simulink model "transfer_function_calculation"  (R2016a)
settings: Solver=VariableStepAuto  StartTime=0.0  StopTime=5  RelTol=1e-3
values from neighbouring files (symbols this model uses):
  a = .7    (= 0.7)    [PM_1_5MW_syn_27.m]
  Flux = 5.8264    [PM_1_5MW_syn_27.m]
  Id_set = 500    [PM_1_5MW_syn_27.m]
  Iq_set = -2200    [PM_1_5MW_syn_27.m]
  L = .0001    (= 0.0001)    [PM_1_5MW_syn_27.m]
  Ld = 0.001575    [PM_1_5MW_syn_27.m]
  Lq = 0.001575    [PM_1_5MW_syn_27.m]
  mn = 60000    [PM_1_5MW_syn_27.m]
  p = 26    [PM_1_5MW_syn_27.m]
  Rs = 0.000821    [PM_1_5MW_syn_27.m]
  Sollkurve_M_Optimum = [0 57121 101549 158670 228485 310994 406196 514092 634681 767965 810425 823386 ... (13 elements, 13x1)]    [Lookup_M_n.mat]
  Sollkurve_nGen_Optimum = [0 5 7 9 11 12 14 16 18 20 20.07 20.2 ... (13 elements, 13x1)]    [Lookup_M_n.mat]
  Speed_set = w_m    (= 2.10172548525)    [PM_1_5MW_syn_27.m]
  Ts_Power = 5.000000000000000e-06    (= 5e-06)    [PM_1_5MW_syn_27.m]
  Vdc = 1200    [PM_1_5MW_syn_27.m]
  Vh = Vm/6*0    (= 0)    [PM_1_5MW_syn_27.m]
undefined symbols (not defined in the file or in its folder): C2, Esw_Erec, Esw_Off, Esw_On, Page_Temp_C
undefined symbols (not defined in the file): Ts_Control, z
libraries: fl_lib x84, powerlib_meascontrol x58, simulink x56, nesl_utility x36, powerlib x33, simulink_extras x11
(part 1 of 6)
settings Model: Creator=Test  LastModifiedBy=Test

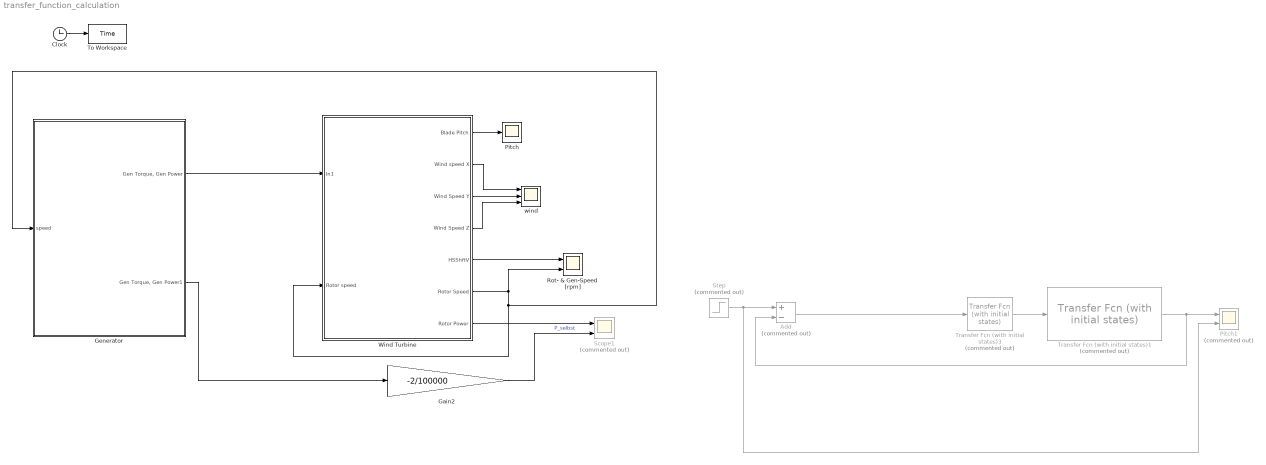
== system transfer_function_calculation ==
  Add : Sum  Commented=on  Inputs=+-
  Clock : Clock
  Gain2 : Gain  Gain=-2/100000
  Generator : Subsystem
  Pitch : Scope
  Pitch1 : Scope  Commented=on  NumInputPorts=2
  Rot- & Gen-Speed [rpm] : Scope  NumInputPorts=2
  Scope1 : Scope  Commented=on  NumInputPorts=2
  Step : Step  Commented=on  SampleTime=0
  To Workspace : ToWorkspace  VariableName=Time  SampleTime=-1
  Transfer Fcn (with initial states)1 : simulink_extras/Additional Linear/Transfer Fcn (with initial states)  Commented=on  N=[6349]  D=[1 10.52 5.213]  X0=0
  Transfer Fcn (with initial states)3 : simulink_extras/Additional Linear/Transfer Fcn (with initial states)  Commented=on  N=[-627e-6 1]*5  D=[627e-6 1]  X0=0
  Wind Turbine : Subsystem
  wind : Scope  NumInputPorts=3
  wires:
  Clock/1 -> To Workspace/1
  Generator/2("Gen Torque, Gen Power1") -> Gain2/1
  Gain2/1 -> Scope1/2  "P_selbst"
  Wind Turbine/6(Rotor Speed) -> Generator/1(speed), Wind Turbine/2(Rotor speed), Rot- & Gen-Speed [rpm]/2
  Generator/1("Gen Torque, Gen Power") -> Wind Turbine/1(In1)
  Wind Turbine/1(Blade Pitch) -> Pitch/1
  Wind Turbine/2(Wind speed X) -> wind/1
  Wind Turbine/3(Wind Speed Y) -> wind/2
  Wind Turbine/4(Wind Speed Z) -> wind/3
  Wind Turbine/7(Rotor Power) -> Scope1/1
  Wind Turbine/5(HSShftV) -> Rot- & Gen-Speed [rpm]/1
  Transfer Fcn (with initial states)1/1 -> Add/2, Pitch1/1
  Step/1 -> Pitch1/2, Add/1
  Add/1 -> Transfer Fcn (with initial states)3/1
  Transfer Fcn (with initial states)3/1 -> Transfer Fcn (with initial states)1/1

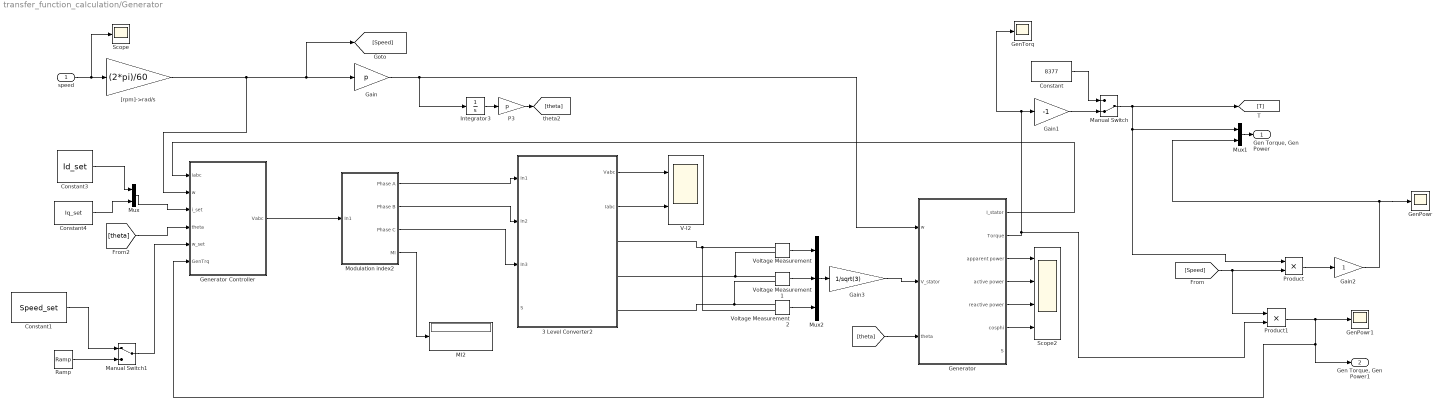
== system transfer_function_calculation/Generator ==
  speed : Inport
  3 Level Converter2 : Subsystem
  Constant : Constant  Value=8377  VectorParams1D=off
  Constant1 : Constant  Value=Speed_set  VectorParams1D=off
  Constant3 : Constant  Value=Id_set
  Constant4 : Constant  Value=Iq_set
  Gain : Gain  Gain=p
  Gain1 : Gain  Gain=-1
  Gain2 : Gain
  Gain3 : Gain  Gain=1/sqrt(3)
  GenPowr : Scope
  GenPowr1 : Scope
  GenTorq : Scope
  "Generator " : Subsystem
  "Generator Controller " : Subsystem
  Integrator3 : Integrator
  MI2 : Display
  Manual Switch : ManualSwitch  CurrentSetting=0
  Manual Switch1 : ManualSwitch
  Modulation index2 : Subsystem
  Mux : Mux  Inputs=2
  Mux1 : Mux  Inputs=2
  Mux2 : Mux  Inputs=3
  P3 : Gain  Gain=p
  Product : Product
  Product1 : Product
  Ramp : simulink/Sources/Ramp  slope=1/60*2*pi/10  start=40  X0=1.831548517042849
  Scope : Scope
  Scope2 : Scope  NumInputPorts=4
  V-I2 : Scope  NumInputPorts=2
  Voltage Measurement : powerlib/Measurements/Voltage Measurement  PhasorSimulation=off  OutputType=Complex  PSBequivalent=0
  Voltage Measurement1 : powerlib/Measurements/Voltage Measurement  PhasorSimulation=off  OutputType=Complex  PSBequivalent=0
  Voltage Measurement2 : powerlib/Measurements/Voltage Measurement  PhasorSimulation=off  OutputType=Complex  PSBequivalent=0
  "[rpm]->rad/s" : Gain  Gain=(2*pi)/60
  "Gen Torque, Gen Power" : Outport
  "Gen Torque, Gen Power1" : Outport  Port=2
  wires:
  speed/1 -> "[rpm]->rad/s"/1, Scope/1
  "Generator "/1("I_stator ") -> "Generator Controller "/1(iabc)
  Constant3/1 -> Mux/1
  "Generator "/5(reactive power) -> Scope2/3
  [theta] -> "Generator Controller "/4(theta)
  Constant4/1 -> Mux/2
  "Generator "/6(cosphi) -> Scope2/4
  "Generator "/3(apparent power) -> Scope2/1
  "Generator "/4(active power) -> Scope2/2
  Constant1/1 -> Manual Switch1/1
  [theta] -> "Generator "/3("theta ")
  Mux/1 -> "Generator Controller "/3(i_set)
  Gain/1 -> "Generator "/1(w), Integrator3/1
  "[rpm]->rad/s"/1 -> "Generator Controller "/2(w), [Speed], Gain/1
  Integrator3/1 -> P3/1
  [Speed] -> Product/2, Product1/1
  Product1/1 -> "Generator Controller "/6(GenTrq), "Gen Torque, Gen Power1"/1, GenPowr1/1
  Mux1/1 -> "Gen Torque, Gen Power"/1
  Product/1 -> Gain2/1
  Constant/1 -> Manual Switch/1
  Gain2/1 -> GenPowr/1, Mux1/2
  "Generator "/2(Torque) -> GenTorq/1, Gain1/1, Product1/2
  Manual Switch/1 -> [T], Mux1/1, Product/1
  Manual Switch1/1 -> "Generator Controller "/5(w_set)
  Ramp/1 -> Manual Switch1/2
  Gain1/1 -> Manual Switch/2
  P3/1 -> [theta]
  3 Level Converter2/2(Iabc) -> V-I2/2
  Modulation index2/1(Phase A) -> 3 Level Converter2/1(In1)
  Modulation index2/2(Phase B) -> 3 Level Converter2/2(In2)
  Modulation index2/3(Phase C) -> 3 Level Converter2/3(In3)
  Modulation index2/4(MI) -> MI2/1
  3 Level Converter2/1(Vabc) -> V-I2/1
  Voltage Measurement/1 -> Mux2/1
  Voltage Measurement1/1 -> Mux2/2
  Voltage Measurement2/1 -> Mux2/3
  Mux2/1 -> Gain3/1
  Gain3/1 -> "Generator "/2("V_stator ")
  "Generator Controller "/1(Vabc) -> Modulation index2/1(In1)
  connections:
  Voltage Measurement/LConn1 -- Voltage Measurement2/LConn2 -- 3 Level Converter2/RConn1
  Voltage Measurement1/LConn1 -- Voltage Measurement/LConn2 -- 3 Level Converter2/RConn2
  Voltage Measurement2/LConn1 -- Voltage Measurement1/LConn2 -- 3 Level Converter2/RConn3

== system transfer_function_calculation/Wind Turbine ==
  In1 : Inport
  Rotor speed : Inport  Port=2
  FAST Nonlinear Wind Turbine : Subsystem  mask(FAST Nonlinear Wind Turbine){}
      mask help: This block contains the FAST S-Function.
      mask init:
      | clear FAST_SFunc
  High-Speed Shaft Brake : Subsystem
  Pitch Controller : Subsystem
  "Turbine Output Scope " : Subsystem
  Yaw Controller : Subsystem
  Blade Pitch : Outport
  Wind speed X : Outport  Port=2
  Wind Speed Y : Outport  Port=3
  Wind Speed Z : Outport  Port=4
  HSShftV : Outport  Port=5
  Rotor Speed : Outport  Port=6
  Rotor Power : Outport  Port=7
  wires:
  Pitch Controller/1(Out1) -> FAST Nonlinear Wind Turbine/3(Blade Pitch Angles (rad))
  Yaw Controller/1(Out1) -> FAST Nonlinear Wind Turbine/2(Yaw Position (rad) and Rate (rad/s))
  High-Speed Shaft Brake/1(Out1) -> FAST Nonlinear Wind Turbine/4(High-Speed Shaft Braking Fraction (-))
  In1/1 -> FAST Nonlinear Wind Turbine/1(Gen. Torque (Nm) and Power (W))
  Rotor speed/1 -> "Turbine Output Scope "/1(Rotor speed)
  FAST Nonlinear Wind Turbine/1(OutData) -> "Turbine Output Scope "/2(In1)
  "Turbine Output Scope "/1(Blade Pitch) -> Blade Pitch/1
  "Turbine Output Scope "/2(Wind speed X) -> Wind speed X/1
  "Turbine Output Scope "/3(Wind Speed Y) -> Wind Speed Y/1
  "Turbine Output Scope "/4(Wind Speed Z) -> Wind Speed Z/1
  "Turbine Output Scope "/5(HSShftV) -> HSShftV/1
  "Turbine Output Scope "/6(Rotor Power) -> Rotor Power/1
  "Turbine Output Scope "/7(Rotor Speed) -> Rotor Speed/1

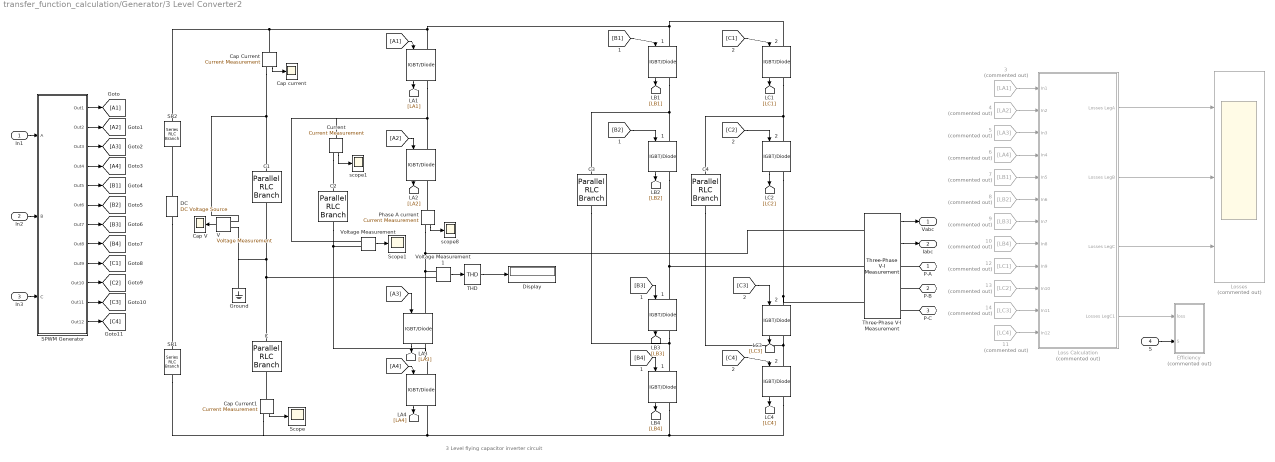
== system transfer_function_calculation/Generator/3 Level Converter2 ==
  note: 3 Level flying capacitor inverter circuit
  In1 : Inport
  In2 : Inport  Port=2
  In3 : Inport  Port=3
  S : Inport  Port=4
  "    " : powerlib/Power Electronics/IGBT//Diode  Ron=1e-3  Rs=1e5  Cs=inf  Measurements=on
  "       " : powerlib/Power Electronics/IGBT//Diode  Ron=1e-3  Rs=1e5  Cs=inf  Measurements=on
  "          " : powerlib/Power Electronics/IGBT//Diode  Ron=1e-3  Rs=1e5  Cs=inf  Measurements=on
  "            " : powerlib/Power Electronics/IGBT//Diode  Ron=1e-3  Rs=1e5  Cs=inf  Measurements=on
  "            1" : powerlib/Power Electronics/IGBT//Diode  Ron=1e-3  Rs=1e5  Cs=inf  Measurements=on
  "            2" : powerlib/Power Electronics/IGBT//Diode  Ron=1e-3  Rs=1e5  Cs=inf  Measurements=on
  "          1" : powerlib/Power Electronics/IGBT//Diode  Ron=1e-3  Rs=1e5  Cs=inf  Measurements=on
  "          2" : powerlib/Power Electronics/IGBT//Diode  Ron=1e-3  Rs=1e5  Cs=inf  Measurements=on
  "       1" : powerlib/Power Electronics/IGBT//Diode  Ron=1e-3  Rs=1e5  Cs=inf  Measurements=on
  "       2" : powerlib/Power Electronics/IGBT//Diode  Ron=1e-3  Rs=1e5  Cs=inf  Measurements=on
  "    1" : powerlib/Power Electronics/IGBT//Diode  Ron=1e-3  Rs=1e5  Cs=inf  Measurements=on
  "    2" : powerlib/Power Electronics/IGBT//Diode  Ron=1e-3  Rs=1e5  Cs=inf  Measurements=on
  " 10" : From  Commented=on  GotoTag=LB4
  " 11" : From  Commented=on  GotoTag=LC4
  " 12" : From  Commented=on  GotoTag=LC1
  " 13" : From  Commented=on  GotoTag=LC2
  " 14" : From  Commented=on  GotoTag=LC3
  " 3" : From  Commented=on  GotoTag=LA1
  " 4" : From  Commented=on  GotoTag=LA2
  " 5" : From  Commented=on  GotoTag=LA3
  " 6" : From  Commented=on  GotoTag=LA4
  " 7" : From  Commented=on  GotoTag=LB1
  " 8" : From  Commented=on  GotoTag=LB2
  " 9" : From  Commented=on  GotoTag=LB3
  C : powerlib/Elements/Parallel RLC Branch  LConnTagsString=a  RConnTagsString=__new0  BranchType=C  Resistance=1  Inductance=1e-3  SetiL0=off  InitialCurrent=0  Capacitance=C2  Setx0=off  InitialVoltage=Vdc/2  Measurements=None
  C1 : powerlib/Elements/Parallel RLC Branch  LConnTagsString=a  RConnTagsString=__new0  BranchType=C  Resistance=1  Inductance=1e-3  SetiL0=off  InitialCurrent=0  Capacitance=C2  Setx0=off  InitialVoltage=Vdc/2  Measurements=None
  C2 : powerlib/Elements/Parallel RLC Branch  LConnTagsString=a  RConnTagsString=__new0  BranchType=C  Resistance=1  Inductance=1e-3  SetiL0=off  InitialCurrent=0  Capacitance=.02  Setx0=off  InitialVoltage=600  Measurements=None
  C3 : powerlib/Elements/Parallel RLC Branch  LConnTagsString=a  RConnTagsString=__new0  BranchType=C  Resistance=1  Inductance=1e-3  SetiL0=off  InitialCurrent=0  Capacitance=.02  Setx0=off  InitialVoltage=0  Measurements=None
  C4 : powerlib/Elements/Parallel RLC Branch  LConnTagsString=a  RConnTagsString=__new0  BranchType=C  Resistance=1  Inductance=1e-3  SetiL0=off  InitialCurrent=0  Capacitance=.02  Setx0=off  InitialVoltage=0  Measurements=Branch voltage
  Cap Current : powerlib/Measurements/Current Measurement  PhasorSimulation=off  OutputType=Complex  PSBequivalent=0
  Cap Current1 : powerlib/Measurements/Current Measurement  PhasorSimulation=off  OutputType=Complex  PSBequivalent=0
  Cap V : Scope
  Cap current : Scope
  Current : powerlib/Measurements/Current Measurement  PhasorSimulation=off  OutputType=Complex  PSBequivalent=0
  DC : powerlib/Electrical Sources/DC Voltage Source  Amplitude=Vdc  Measurements=None
  Display : Display
  Efficiency : Subsystem  Commented=on
  Ground : powerlib/Elements/Ground  LConnTagsString=a
  Loss Calculation : Subsystem  Commented=on
      mask Display: image('C:\Users\Test\Desktop\inverter losses\loss.jpg');
  Losses : Scope  Commented=on  NumInputPorts=3
  "Phase A current " : powerlib/Measurements/Current Measurement  PhasorSimulation=off  OutputType=Complex  PSBequivalent=0
  SPWM Generator : Subsystem
  SR1 : powerlib/Elements/Series RLC Branch  LConnTagsString=__new0  RConnTagsString=__new0  BranchType=R  Resistance=.02  Inductance=L  SetiL0=off  InitialCurrent=0  Capacitance=1e-6  Setx0=off  InitialVoltage=0  Measurements=None
  SR2 : powerlib/Elements/Series RLC Branch  LConnTagsString=__new0  RConnTagsString=__new0  BranchType=R  Resistance=.02  Inductance=L  SetiL0=off  InitialCurrent=0  Capacitance=1e-6  Setx0=off  InitialVoltage=0  Measurements=None
  Scope : Scope
  Scope1 : Scope
  THD : powerlib_meascontrol/Measurements/THD  Freq=60  Ts=0
  Three-Phase V-I Measurement : powerlib/Measurements/Three-Phase V-I Measurement  VoltageMeasurement=phase-to-ground  SetLabelV=off  LabelV=Vabc  Vpu=off  VpuLL=off  CurrentMeasurement=yes  SetLabelI=off  LabelI=Iabc  Ipu=off  Pbase=100e6  Vbase=500e3  OutputType=Complex  PhasorSimulation=off  PSBequivalent=0
  V : powerlib/Measurements/Voltage Measurement  PhasorSimulation=off  OutputType=Complex  PSBequivalent=0
  Voltage Measurement : powerlib/Measurements/Voltage Measurement  PhasorSimulation=off  OutputType=Complex  PSBequivalent=0
  Voltage Measurement1 : powerlib/Measurements/Voltage Measurement  PhasorSimulation=off  OutputType=Complex  PSBequivalent=0
  scope1 : Scope
  scope8 : Scope
  P-A : PMIOPort  Port=1  Side=Right
  P-B : PMIOPort  Port=2  Side=Right
  P-C : PMIOPort  Port=3  Side=Right
  Vabc : Outport
  Iabc : Outport  Port=2
  wires:
  In1/1 -> SPWM Generator/1(A)
  SPWM Generator/2(Out2) -> [A2]
  SPWM Generator/5(Out5) -> [B1]
  SPWM Generator/8(Out8) -> [B4]
  SPWM Generator/9(Out9) -> [C1]
  In2/1 -> SPWM Generator/2(B)
  SPWM Generator/3(Out3) -> [A3]
  SPWM Generator/6(Out6) -> [B2]
  SPWM Generator/7(Out7) -> [B3]
  SPWM Generator/1(Out1) -> [A1]
  SPWM Generator/4(Out4) -> [A4]
  In3/1 -> SPWM Generator/3(C)
  SPWM Generator/12(Out12) -> [C4]
  SPWM Generator/10(Out10) -> [C2]
  SPWM Generator/11(Out11) -> [C3]
  Three-Phase V-I Measurement/2 -> Iabc/1
  Three-Phase V-I Measurement/1 -> Vabc/1
  [A2] -> "    "/1
  [A1] -> "            "/1
  [A3] -> "       "/1
  [A4] -> "          "/1
  [B1] -> "            1"/1
  [B2] -> "    1"/1
  [B3] -> "       1"/1
  [B4] -> "          1"/1
  [C1] -> "            2"/1
  [C2] -> "    2"/1
  [C3] -> "       2"/1
  [C4] -> "          2"/1
  "Phase A current "/1 -> scope8/1
  Cap Current/1 -> Cap current/1
  Current/1 -> scope1/1
  "            "/1 -> [LA1]
  "    "/1 -> [LA2]
  "       "/1 -> [LA3]
  "          "/1 -> [LA4]
  "            1"/1 -> [LB1]
  "    1"/1 -> [LB2]
  "       1"/1 -> [LB3]
  "          1"/1 -> [LB4]
  "            2"/1 -> [LC1]
  "    2"/1 -> [LC2]
  "       2"/1 -> [LC3]
  "          2"/1 -> [LC4]
  " 3"/1 -> Loss Calculation/1(In1)
  " 4"/1 -> Loss Calculation/2(In2)
  " 5"/1 -> Loss Calculation/3(In3)
  " 6"/1 -> Loss Calculation/4(In4)
  " 7"/1 -> Loss Calculation/5(In5)
  " 8"/1 -> Loss Calculation/6(In6)
  " 9"/1 -> Loss Calculation/7(In7)
  " 10"/1 -> Loss Calculation/8(In8)
  " 12"/1 -> Loss Calculation/9(In9)
  " 13"/1 -> Loss Calculation/10(In10)
  " 14"/1 -> Loss Calculation/11(In11)
  " 11"/1 -> Loss Calculation/12(In12)
  Loss Calculation/1(Losses LegA) -> Losses/1
  Loss Calculation/2(Losses LegB) -> Losses/2
  Loss Calculation/3(Losses LegC) -> Losses/3
  V/1 -> Cap V/1
  Cap Current1/1 -> Scope/1
  Loss Calculation/4(Losses LegC1) -> Efficiency/1(loss)
  Voltage Measurement/1 -> Scope1/1
  Voltage Measurement1/1 -> THD/1
  THD/1 -> Display/1
  S/1 -> Efficiency/2("S ")
  connections:
  P-B/RConn1 -- Three-Phase V-I Measurement/RConn2
  P-C/RConn1 -- Three-Phase V-I Measurement/RConn3
  "            "/RConn1 -- Current/LConn1 -- Voltage Measurement/LConn1 -- "    "/LConn1
  "          1"/RConn1 -- "          2"/RConn1 -- Cap Current1/RConn1 -- SR1/RConn1 -- "          "/RConn1
  C2/RConn1 -- Voltage Measurement/LConn2 -- "          "/LConn1 -- "       "/RConn1
  "    1"/RConn1 -- Three-Phase V-I Measurement/LConn2 -- "       1"/LConn1
  "       1"/RConn1 -- C3/RConn1 -- "          1"/LConn1
  "            1"/RConn1 -- "    1"/LConn1 -- C3/LConn1
  C/LConn1 -- Voltage Measurement1/LConn2 -- V/LConn2 -- Ground/LConn1 -- C1/RConn1
  Three-Phase V-I Measurement/LConn1 -- Voltage Measurement1/LConn1 -- "       "/LConn1 -- "Phase A current "/RConn1
  "            2"/RConn1 -- "    2"/LConn1 -- C4/LConn1
  C4/RConn1 -- "       2"/RConn1 -- "          2"/LConn1
  "    2"/RConn1 -- Three-Phase V-I Measurement/LConn3 -- "       2"/LConn1
  P-A/RConn1 -- Three-Phase V-I Measurement/RConn1
  "Phase A current "/LConn1 -- "    "/RConn1
  Cap Current/RConn1 -- C1/LConn1 -- V/LConn1
  Current/RConn1 -- C2/LConn1
  DC/RConn1 -- SR2/RConn1
  DC/LConn1 -- SR1/LConn1
  "            2"/LConn1 -- "            1"/LConn1 -- SR2/LConn1 -- Cap Current/LConn1 -- "            "/LConn1
  Cap Current1/LConn1 -- C/RConn1

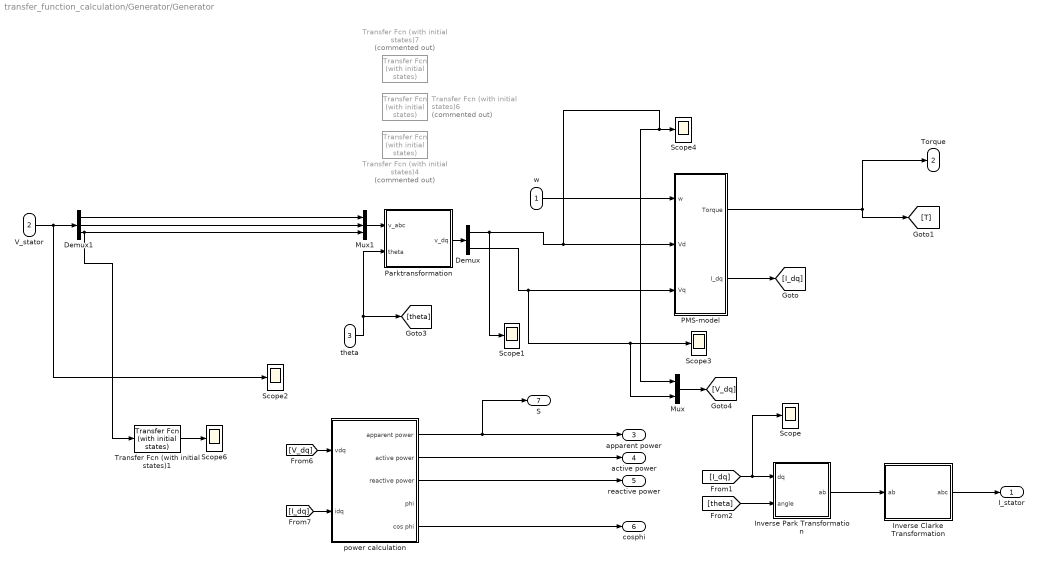
== system transfer_function_calculation/Generator/Generator  ==
  w : Inport
  "V_stator " : Inport  Port=2
  "theta " : Inport  Port=3
  Demux : Demux  Outputs=2
  Demux1 : Demux  Outputs=3
  Inverse Clarke Transformation : Subsystem
  Inverse Park Transformation : Subsystem
  Mux : Mux  Inputs=2
  Mux1 : Mux  Inputs=3
  PMS-model : Subsystem
  Parktransformation : Subsystem
  Scope{,1..4,6} (6 alike) : Scope
  Transfer Fcn (with initial states)1 : simulink_extras/Additional Linear/Transfer Fcn (with initial states)  N=[1]  D="[.01  1]"  X0=0
  Transfer Fcn (with initial states)4 : simulink_extras/Additional Linear/Transfer Fcn (with initial states)  Commented=on  N=[1]  D="[.01  1]"  X0=0
  Transfer Fcn (with initial states)6 : simulink_extras/Additional Linear/Transfer Fcn (with initial states)  Commented=on  N=[1]  D="[.01  1]"  X0=0
  Transfer Fcn (with initial states)7 : simulink_extras/Additional Linear/Transfer Fcn (with initial states)  Commented=on  N=[1]  D="[.01  1]"  X0=0
  power calculation : Subsystem
  "I_stator " : Outport
  Torque : Outport  Port=2
  apparent power : Outport  Port=3
  active power : Outport  Port=4
  reactive power : Outport  Port=5
  cosphi : Outport  Port=6
  S : Outport  Port=7
  wires:
  PMS-model/2(I_dq) -> [I_dq]
  PMS-model/1(Torque) -> [T], Torque/1
  "theta "/1 -> Parktransformation/2(theta), [theta]
  Parktransformation/1(v_dq) -> Demux/1
  w/1 -> PMS-model/1(w)
  Inverse Park Transformation/1(ab) -> Inverse Clarke Transformation/1(ab)
  [I_dq] -> Scope/1, Inverse Park Transformation/1(dq)
  Inverse Clarke Transformation/1(abc) -> "I_stator "/1
  [theta] -> Inverse Park Transformation/2(angle)
  [V_dq] -> power calculation/1(vdq)
  [I_dq] -> power calculation/2(idq)
  power calculation/3(reactive power) -> reactive power/1
  power calculation/2(active power) -> active power/1
  power calculation/1(apparent power) -> S/1, apparent power/1
  power calculation/5(cos phi) -> cosphi/1
  "V_stator "/1 -> Demux1/1, Scope2/1
  Demux/2 -> Mux/2, Scope3/1, PMS-model/3(Vq)
  Demux/1 -> Scope1/1, Mux/1, Scope4/1, PMS-model/2(Vd)
  Mux/1 -> [V_dq]
  Demux1/3 -> Mux1/3, Transfer Fcn (with initial states)1/1
  Mux1/1 -> Parktransformation/1(v_abc)
  Transfer Fcn (with initial states)1/1 -> Scope6/1
  ? -> Transfer Fcn (with initial states)4/1
  ? -> Transfer Fcn (with initial states)7/1
  ? -> Transfer Fcn (with initial states)6/1
  Demux1/1 -> Mux1/1
  Demux1/2 -> Mux1/2

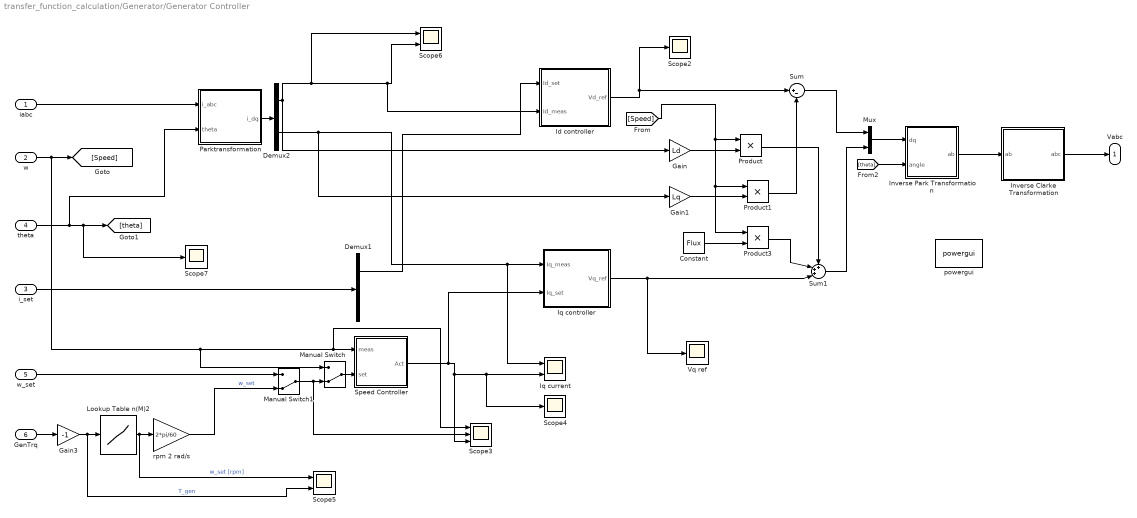
== system transfer_function_calculation/Generator/Generator Controller  ==
  iabc : Inport
  w : Inport  Port=2
  i_set : Inport  Port=3
  theta : Inport  Port=4
  w_set : Inport  Port=5
  GenTrq : Inport  Port=6
  Constant : Constant  Value=Flux
  Demux1 : Demux  Outputs=2
  Demux2 : Demux  Outputs=2
  Gain : Gain  Gain=Ld
  Gain1 : Gain  Gain=Lq
  Gain3 : Gain  Gain=-1
  Id controller : Subsystem
  Inverse Clarke Transformation : Subsystem
  Inverse Park Transformation : Subsystem
  Iq controller : Subsystem
  Iq current : Scope  NumInputPorts=2
  Lookup Table n(M)2 : Lookup_n-D  NumberOfTableDimensions=1  BreakpointsForDimension1=Sollkurve_M_Optimum  Table=Sollkurve_nGen_Optimum  InternalRulePriority=Speed  RndMeth=Simplest  InputSameDT=on
  Manual Switch : ManualSwitch  CurrentSetting=0
  Manual Switch1 : ManualSwitch  CurrentSetting=0
  Mux : Mux  Inputs=2
  Parktransformation : Subsystem
  Product : Product
  Product1 : Product
  Product3 : Product
  Scope2 : Scope
  Scope3 : Scope  NumInputPorts=3
  Scope4 : Scope
  Scope5 : Scope  NumInputPorts=2
  Scope6 : Scope  NumInputPorts=2
  Scope7 : Scope
  Speed Controller : Subsystem
  Sum : Sum  Inputs=|+-
  Sum1 : Sum  Inputs=+++|
  Vq ref : Scope
  powergui : powerlib/powergui  Priority=1  SimulationMode=Discrete  SolverType=Tustin/Backward Euler (TBE)  SampleTime=50e-6  frequency=60  SPID=off  DisableSnubberDevices=off  DisableRonSwitches=off  DisableVfSwitches=off  SwTol=0  DisplayEquations=off  Interpol=off  ExternalGateDelay=off  methode=off  Ts=100  FunctionMessages=off  echomessages=off  HookPort=off  EnableUseOfTLC=off  x0status=blocks  frequencyindice=0  Pbase=100e6  ErrMax=1e-4  Iterations=50  UnitsV=kV  UnitsW=MW  buscounter=0  RestoreLinks=warning  ResistiveCurrentMeasurement=off  Frange=[0:2:500]  Ylog=off  Xlog=on  ShowGrid=off  save=off  variable=ZData  structure=vq  ZoomFFT=off  StartTime=0.02  cycles=10  DisplayStyle=5  fundamental=270  FreqAxis=off  MaxFrequency=4000  frequencyindicesteady=1  RmsSteady=1  display=off
  rpm 2 rad/s : Gain  Gain=2*pi/60
  Vabc : Outport
  wires:
  iabc/1 -> Parktransformation/1(i_abc)
  i_set/1 -> Demux1/1
  Demux1/1 -> Id controller/1(Id_set)
  Gain/1 -> Product/2
  Gain1/1 -> Product1/2
  Product1/1 -> Sum/2
  Product/1 -> Sum1/1
  Inverse Park Transformation/1(ab) -> Inverse Clarke Transformation/1(ab)
  Inverse Clarke Transformation/1(abc) -> Vabc/1
  Sum/1 -> Mux/1
  Sum1/1 -> Mux/2
  Mux/1 -> Inverse Park Transformation/1(dq)
  theta/1 -> Parktransformation/2(theta), Scope7/1, [theta]
  [theta] -> Inverse Park Transformation/2(angle)
  Iq controller/1(Vq_ref) -> Vq ref/1, Sum1/3
  Constant/1 -> Product3/2
  Product3/1 -> Sum1/2
  w/1 -> Scope3/1, Speed Controller/1(meas), Manual Switch/1, [Speed]
  Manual Switch/1 -> Speed Controller/2(set)
  Speed Controller/1(Act) -> Iq controller/2(Iq_set), Scope4/1, Iq current/2, Scope3/3
  Gain3/1 -> Scope5/2, Lookup Table n(M)2/1  "T_gen"
  rpm 2 rad/s/1 -> Manual Switch1/2  "w_set"
  w_set/1 -> Manual Switch1/1
  Manual Switch1/1 -> Scope3/2, Manual Switch/2
  Lookup Table n(M)2/1 -> Scope5/1, rpm 2 rad/s/1  "w_set [rpm]"
  GenTrq/1 -> Gain3/1
  Parktransformation/1(i_dq) -> Demux2/1
  Id controller/1(Vd_ref) -> Sum/1, Scope2/1
  Demux2/2 -> Iq current/1, Iq controller/1(Iq_meas), Gain1/1
  Demux2/1 -> Id controller/2(Id_meas), Scope6/2, Scope6/1, Gain/1
  [Speed] -> Product/1, Product3/1, Product1/1

== system transfer_function_calculation/Generator/Modulation index2 ==
  In1 : Inport
  "   " : Demux  Outputs=2
  Cartesian to Polar : simulink_extras/Transformations/Cartesian to Polar
  Clarke transformation : Subsystem
  Demux : Demux  Outputs=3
  Divide : Product  Inputs=*/
  Gain : Gain  Gain=mn
  Magnitude of triangular wave : Constant  Value=a*2
  Scope1 : Scope
  Scope2 : Scope  NumInputPorts=2
  Scope4 : Scope  NumInputPorts=2
  Space vector magnitude : Display
  Space vector phase : Display
  Phase A : Outport
  Phase B : Outport  Port=2
  Phase C : Outport  Port=3
  MI : Outport  Port=4
  wires:
  Demux/3 -> Phase C/1
  Demux/2 -> Phase B/1
  Demux/1 -> Phase A/1
  "   "/1 -> Cartesian to Polar/1
  "   "/2 -> Cartesian to Polar/2
  Cartesian to Polar/1 -> Divide/1, Space vector magnitude/1, Scope4/1
  Clarke transformation/1(Out1) -> Scope2/2, "   "/1
  Cartesian to Polar/2 -> Space vector phase/1, Scope4/2
  Magnitude of triangular wave/1 -> Divide/2
  Divide/1 -> MI/1
  In1/1 -> Gain/1
  Gain/1 -> Clarke transformation/1(In1), Scope2/1, Scope1/1, Demux/1

== system transfer_function_calculation/Wind Turbine/FAST Nonlinear Wind Turbine ==
  Gen. Torque (Nm) and Power (W) : Inport
  Yaw Position (rad) and Rate (rad/s) : Inport  Port=2
  Blade Pitch Angles (rad) : Inport  Port=3
  High-Speed Shaft Braking Fraction (-) : Inport  Port=4
  Mux1 : Mux
  S-Function : S-Function  FunctionName=FAST_SFunc  Parameters=FAST_InputFileName, TMax, 0  SFunctionDeploymentMode=off  EnableBusSupport=off
  Signal Specification1 : SignalSpecification  OutDataTypeStr=double  Dimensions=2
  Signal Specification2 : SignalSpecification  OutDataTypeStr=double  Dimensions=2
  OutData : Outport
  wires:
  Gen. Torque (Nm) and Power (W)/1 -> Signal Specification1/1
  S-Function/1 -> OutData/1
  Mux1/1 -> S-Function/1
  Blade Pitch Angles (rad)/1 -> Mux1/3
  Yaw Position (rad) and Rate (rad/s)/1 -> Signal Specification2/1
  Signal Specification1/1 -> Mux1/1
  Signal Specification2/1 -> Mux1/2
  High-Speed Shaft Braking Fraction (-)/1 -> Mux1/4

== system transfer_function_calculation/Wind Turbine/High-Speed Shaft Brake ==
  High-Speed Shaft Braking Fraction : Constant  Value=100
  Out1 : Outport
  wires:
  High-Speed Shaft Braking Fraction/1 -> Out1/1

== system transfer_function_calculation/Wind Turbine/Pitch Controller ==
  Blade Pitch Angles : Constant  Value=ones(1,3)'
  Pitch-winkel : Gain  Gain=20
  dergree2rad : Gain  Gain=2*pi/360
  Out1 : Outport
  wires:
  Blade Pitch Angles/1 -> Pitch-winkel/1
  Pitch-winkel/1 -> dergree2rad/1
  dergree2rad/1 -> Out1/1

== system transfer_function_calculation/Wind Turbine/Turbine Output Scope  ==
  Rotor speed : Inport
  In1 : Inport  Port=2
  Demux : Demux  Outputs=34
  GBRatio : Gain  Gain=87.965
  GBRatio [rpm] : Gain  Gain=87.965
  Gen Torqe : Scope  NumInputPorts=2
  Product : Product
  Product1 : Product
  Rot- & Gen-Pwr : Scope  NumInputPorts=4
  Rot- & Gen-Speed [rad/s] : Scope  NumInputPorts=2
  Rot- & Gen-Speed [rpm] : Scope  NumInputPorts=2
  Scope : Scope
  Scope2 : Scope
  qdotdot_out : ToWorkspace  VariableName=OutData  SampleTime=-1
  rpm to rad/s : Gain  Gain=2*pi/60
  rpm to rad/s1 : Gain  Gain=2*pi/60
  Blade Pitch : Outport
  Wind speed X : Outport  Port=2
  Wind Speed Y : Outport  Port=3
  Wind Speed Z : Outport  Port=4
  HSShftV : Outport  Port=5
  Rotor Power : Outport  Port=6
  Rotor Speed : Outport  Port=7
  wires:
  Demux/19 -> Rot- & Gen-Pwr/2  "RotPwr    [kW]"
  Demux/32 -> Gen Torqe/2, HSShftV/1, Rot- & Gen-Speed [rpm]/2, rpm to rad/s1/1  "HSShftV    [rpm]"
  Demux/5 -> Rotor Speed/1, rpm to rad/s/1  "RotSpeed  [rpm]"
  Product/1 -> Rotor Power/1, Rot- & Gen-Pwr/1  "RotPwr_selbs [kW]"
  rpm to rad/s/1 -> Scope/1, GBRatio/1, Product/2  "RotSpeed  [rad/s]"
  In1/1 -> qdotdot_out/1, Demux/1
  Demux/34 -> Rot- & Gen-Pwr/3  "GenPwr    [kW]"
  Demux/33 -> Gen Torqe/1, Product1/1  "GenTq [kN/m]"
  Demux/18 -> Product/1, Scope2/1  "RotTorq   [kN-m]"
  GBRatio [rpm]/1 -> Rot- & Gen-Speed [rpm]/1  "RotSpeed * GBRatio [rpm]"
  Demux/3 -> Wind Speed Y/1  "Wind1VelY [m/s]"
  Product1/1 -> Rot- & Gen-Pwr/4  "GenPwr_selbst [kW]"
  Demux/2 -> Wind speed X/1  "Wind1VelX [m/s]"
  GBRatio/1 -> Rot- & Gen-Speed [rad/s]/1
  Demux/6 -> Blade Pitch/1  "BldPitch1"
  rpm to rad/s1/1 -> Rot- & Gen-Speed [rad/s]/2, Product1/2  "HSShftV    [rad/s]"
  Demux/4 -> Wind Speed Z/1  "Wind1VelZ [m/s]"
  Rotor speed/1 -> GBRatio [rpm]/1

== system transfer_function_calculation/Wind Turbine/Yaw Controller ==
  Mux : Mux  Inputs=2
  Yaw Position : Constant  Value=0
  Yaw rate : Constant  Value=0
  Out1 : Outport
  wires:
  Mux/1 -> Out1/1
  Yaw Position/1 -> Mux/1
  Yaw rate/1 -> Mux/2

== system transfer_function_calculation/Generator/3 Level Converter2/Efficiency ==
  loss : Inport
  "S " : Inport  Port=2
  Constant2 : Constant
  Divide : Product  Inputs=/*
  Scope4 : Scope
  Sum1 : Sum  Inputs=|-+
  wires:
  loss/1 -> Divide/2
  Divide/1 -> Sum1/1
  Constant2/1 -> Sum1/2
  Sum1/1 -> Scope4/1
  "S "/1 -> Divide/1
